simulink model "DC_motor_control_simulink"  (R2025b)
settings: Solver=VariableStepAuto  StartTime=0.0  StopTime=10.0  RelTol=1e-3
values from neighbouring files (symbols this model uses):
  B = 0.1    [DC_motor_control.m]
  J = 0.01    [DC_motor_control.m]
  Ke = 0.01    [DC_motor_control.m]
  Kt = 0.01    [DC_motor_control.m]
  L = 0.5    [DC_motor_control.m]
  R = 1    [DC_motor_control.m]
settings Model: Creator=leonard  LastModifiedBy=leonard

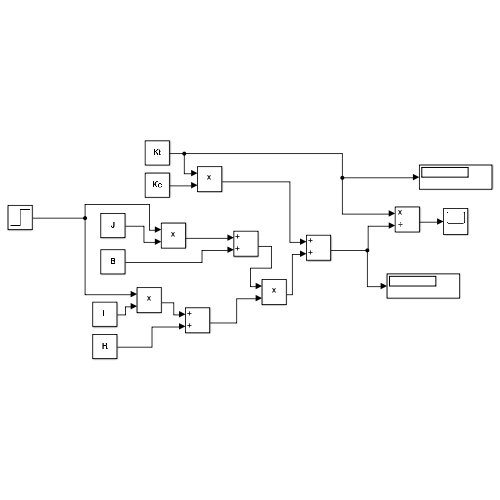
[thumbnail: Simulink's stored preview of the top-level diagram]
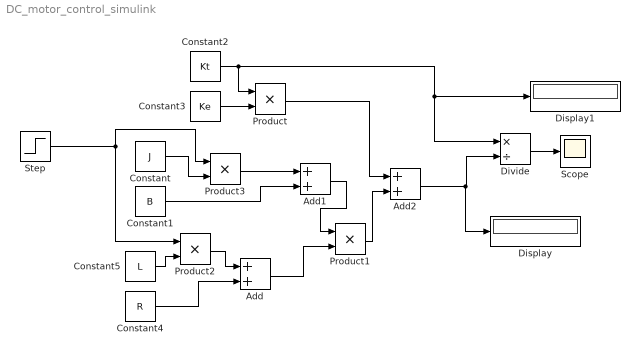
== system DC_motor_control_simulink ==
  Add : Sum
  Add1 : Sum
  Add2 : Sum
  Constant : Constant  Value=J
  Constant1 : Constant  Value=B
  Constant2 : Constant  Value=Kt
  Constant3 : Constant  Value=Ke
  Constant4 : Constant  Value=R
  Constant5 : Constant  Value=L
  Display : Display
  Display1 : Display
  Divide : Product  Inputs=*/
  Product{,1..3} (4 alike) : Product
  Scope : Scope
      settings: ActiveDisplayYMinimum=0.046947729759856657  ActiveDisplayYMaximum=0.10984961249827824
  Step : Step  SampleTime=0
  wires:
  Constant1/1 -> Add1/2
  Constant2/1 -> Product/1, Divide/1, Display1/1
  Add1/1 -> Product1/1
  Product/1 -> Add2/1
  Add2/1 -> Display/1, Divide/2
  Constant3/1 -> Product/2
  Product1/1 -> Add2/2
  Add/1 -> Product1/2
  Constant4/1 -> Add/2
  Product2/1 -> Add/1
  Constant5/1 -> Product2/2
  Step/1 -> Product2/1, Product3/1
  Product3/1 -> Add1/1
  Constant/1 -> Product3/2
  Divide/1 -> Scope/1
